simulink model "m05_target_model"  (R2021b)
settings: Solver=FixedStepAuto  StartTime=0.0  StopTime=inf  FixedStep=Ts  RelTol=1e-3  EnableMultiTasking=on
InitFcn:
  | m04_design_script
values from neighbouring files (symbols this model uses):
  Ts = 0.001    [m03_linearization_script.m]    (also in openLoopAnalysis.m)
libraries: arduinolib x4, cstblocks x2, dspsigops x1, svdutilitieslib x1
settings Model: ExtModeTrigDuration=2  Creator=s269684  LastModifiedBy=s269684
settings OptimizationCC: EnhancedBackFolding=on  PassReuseOutputArgsThreshold=0  MaxStackSize=64  OptimizeBlockOrder=speed  DifferentSizesBufferReuse=on  OptimizationCustomize=off
settings DebuggingCC: ParameterTunabilityLossMsg=error
settings HardwareCC: ProdBitPerInt=16  ProdBitPerPointer=16  ProdBitPerSizeT=16  ProdBitPerPtrDiffT=16  ProdLargestAtomicFloat=None  ProdWordSize=8  ProdHWDeviceType=Atmel->AVR  UseEmbeddedCoderFeatures=off  UseSimulinkCoderFeatures=off
settings SFSimCC: MATLABDynamicMemAlloc=off
settings RTWCC: Description=Embedded Coder  SystemTargetFile=ert.tlc  HardwareBoard=Arduino Uno  TemplateMakefile=ert_default_tmf  Toolchain=Arduino AVR  BuildConfiguration=Faster Runs
settings CodeAppCC: ForceParamTrailComments=on  OperatorAnnotations=on
settings ERTTargetCC: ERTCustomFileBanners=off  SupportContinuousTime=on  SupportNonInlinedSFcns=on  RemoveResetFunc=off  SupportVariableSizeSignals=on  ModelStepFunctionPrototypeControlCompliant=off  ExtModeStaticAllocSize=250

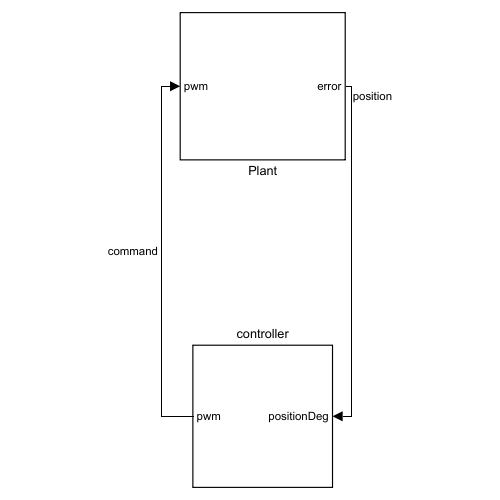
[thumbnail: Simulink's stored preview of the top-level diagram]
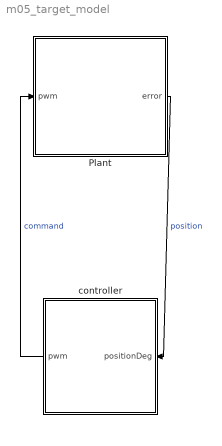
== system m05_target_model ==
  Plant : Subsystem
  controller : Subsystem
  wires:
  Plant/1(error) -> controller/1(positionDeg)  "position"
  controller/1(pwm) -> Plant/1(pwm)  "command"

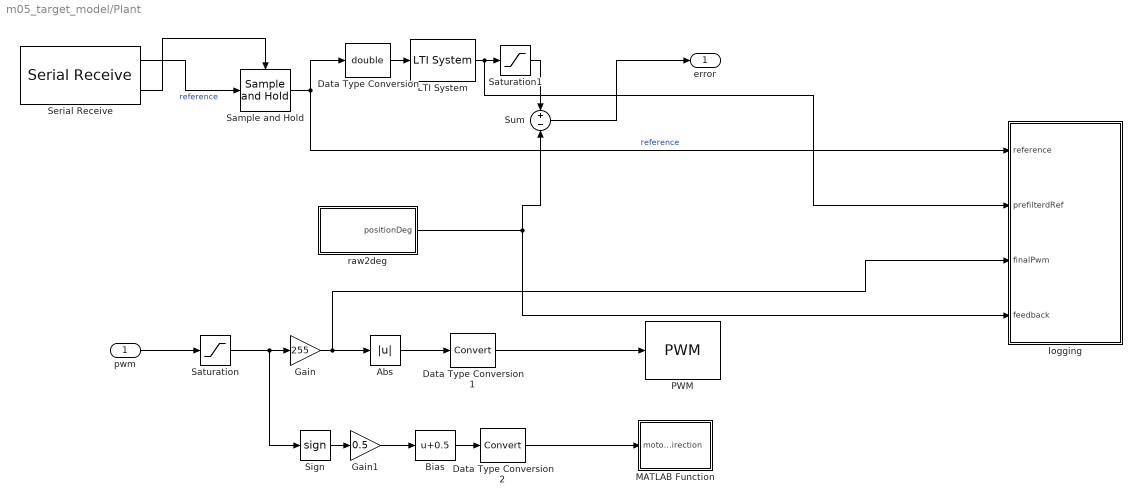
== system m05_target_model/Plant ==
  pwm : Inport
  Abs : Abs
  Bias : Bias  Bias=0.5
  Data Type Conversion : DataTypeConversion  OutDataTypeStr=double
  Data Type Conversion1 : DataTypeConversion
  Data Type Conversion2 : DataTypeConversion
  Gain : Gain  Gain=255
  Gain1 : Gain  Gain=0.5
  LTI System : cstblocks/LTI System  sys=Qd  IC=[]
  MATLAB Function : MATLAB Function  TreatAsAtomicUnit=on
  PWM : arduinolib/PWM  pinNumber=6  frequencyType=Default  desiredFrequency=490.2  achievableFrequency=490.2
  Sample and Hold : dspsigops/Sample and Hold  trig=Rising edge  initCond=0  latchinput=off
  Saturation : Saturate  UpperLimit=1  LowerLimit=-1
  Saturation1 : Saturate  UpperLimit=160  LowerLimit=20
  Serial Receive : arduinolib/Serial Receive  isARMArch=off  portNumber=0  DataType=uint8  Datalength=1  SampleTime=Ts  showOutStatus=on  blockPlatform=arduino
      settings: SourceProductBaseCode=ARDUINO
  Sign : Signum
  Sum : Sum  Inputs=+-
  logging : Subsystem
  raw2deg : Subsystem
  error : Outport
  wires:
  Data Type Conversion/1 -> LTI System/1
  Abs/1 -> Data Type Conversion1/1
  Gain1/1 -> Bias/1
  Data Type Conversion2/1 -> MATLAB Function/1(motorDirection)
  Bias/1 -> Data Type Conversion2/1
  pwm/1 -> Saturation/1
  Sign/1 -> Gain1/1
  Data Type Conversion1/1 -> PWM/1
  Saturation/1 -> Sign/1, Gain/1
  Sum/1 -> error/1
  Sample and Hold/1 -> logging/1(reference), Data Type Conversion/1  "reference"
  Gain/1 -> logging/3(finalPwm), Abs/1
  raw2deg/1(positionDeg) -> Sum/2, logging/4(feedback)
  Saturation1/1 -> Sum/1
  Serial Receive/2 -> Sample and Hold/Trigger
  Serial Receive/1 -> Sample and Hold/1  "reference"
  LTI System/1 -> logging/2(prefilterdRef), Saturation1/1

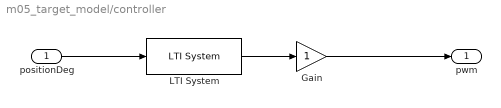
== system m05_target_model/controller ==
  positionDeg : Inport
  Gain : Gain
  LTI System : cstblocks/LTI System  sys=Cd  IC=[]
  pwm : Outport
  wires:
  positionDeg/1 -> LTI System/1
  Gain/1 -> pwm/1
  LTI System/1 -> Gain/1

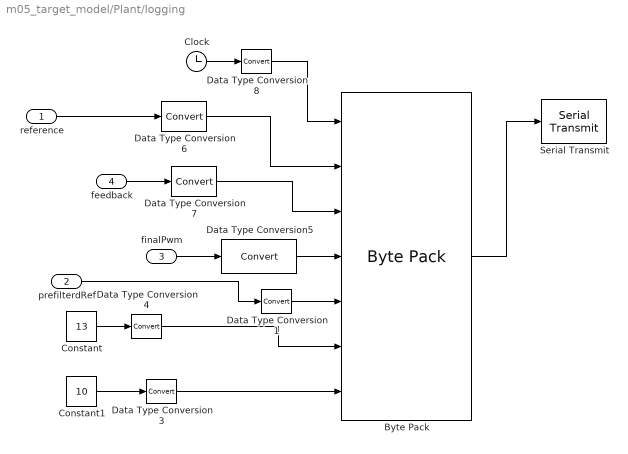
== system m05_target_model/Plant/logging ==
  reference : Inport
  prefilterdRef : Inport  Port=2
  finalPwm : Inport  Port=3
  feedback : Inport  Port=4
  Byte Pack : svdutilitieslib/Byte Pack  maskPackedDataType=uint8  datatypes={'single' , 'single', 'single', 'single','single', 'uint8', 'uint8'}  byteAlign=1  blockPlatform=arduinoert
      settings: SourceProductBaseCode=ANDROID,ARDUINO,ML_ARDUINO,ECCORTEXA,ECCORTEXR,SC_BEAGLEBONE_BLUE,EC_FREEDOM_BOARD,EC_FRDM_K64F,INTEL_BLOCKSET,MICROBIT,NUCLEO,NVIDIA,PX4AUTOPILOTS,RASPPIIO,STMICRODIS,TIC2000,XILINX_BLOCKSET
  Clock : Clock
  Constant : Constant  Value=13
  Constant1 : Constant  Value=10
  Data Type Conversion{1,3..8} (7 alike) : DataTypeConversion
  Serial Transmit : arduinolib/Serial Transmit  portNumber=0  sendmode=write  sendformat=Decimal  floatprecision=2  blockPlatform=arduino
  wires:
  finalPwm/1 -> Data Type Conversion5/1
  Data Type Conversion8/1 -> Byte Pack/1
  Data Type Conversion6/1 -> Byte Pack/2
  feedback/1 -> Data Type Conversion7/1
  Clock/1 -> Data Type Conversion8/1
  Data Type Conversion7/1 -> Byte Pack/3
  reference/1 -> Data Type Conversion6/1
  Byte Pack/1 -> Serial Transmit/1
  Constant1/1 -> Data Type Conversion3/1
  Data Type Conversion5/1 -> Byte Pack/4
  Constant/1 -> Data Type Conversion4/1
  Data Type Conversion3/1 -> Byte Pack/7
  Data Type Conversion4/1 -> Byte Pack/6
  prefilterdRef/1 -> Data Type Conversion1/1
  Data Type Conversion1/1 -> Byte Pack/5

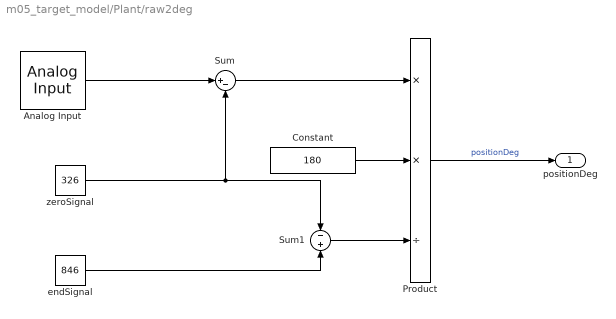
== system m05_target_model/Plant/raw2deg ==
  Analog Input : arduinolib/Analog Input  pinNumber=1  ReadResultsOnly=off  ConversionTriggerSource=Software  ExternalTriggerType=uint32( 0 )  OutputDataType=uint16  EnableConversionCompleteNotify=off  EnableOuputStatus=off  SampleTime=-1  blockPlatform=arduino
  Constant : Constant  Value=180
  Product : Product  Inputs=**/
  Sum : Sum  Inputs=|+-
  Sum1 : Sum  Inputs=-+
  endSignal : Constant  Value=846
  zeroSignal : Constant  Value=326
  positionDeg : Outport
  wires:
  Sum1/1 -> Product/3
  Analog Input/1 -> Sum/1
  zeroSignal/1 -> Sum1/1, Sum/2
  endSignal/1 -> Sum1/2
  Sum/1 -> Product/1
  Constant/1 -> Product/2
  Product/1 -> positionDeg/1  "positionDeg"

== matlab function m05_target_model/Plant/MATLAB Function ==
  data: motorDirection input
function fcn(motorDirection)
persistent arduinoObj;
directionPin = "A0";
if (isempty(arduinoObj))
    arduinoObj = arduino();
    arduinoObj.configurePin(directionPin , "DigitalOutput");
end

arduinoObj.writeDigitalPin(directionPin, motorDirection)
end
